simulink model "schema4"  (R2020b)
settings: Solver=VariableStepAuto  StartTime=0.0  StopTime=10.0  RelTol=1e-3
values from neighbouring files (symbols this model uses):
  DenC = [1]    [TP2.m]    (also in ptschema2.m; ptschema3.m)
  DenG = [1/(16.89*50) 1/16.89 0]    [TP2.m]    (also in ptschema2.m = [1/(16.89*50)  1/16.89 0]; ptschema3.m)
  NumC = [1]    [TP2.m]    (also in ptschema2.m; ptschema3.m)
  NumG = [1]    [TP2.m]    (also in ptschema2.m; ptschema3.m)
settings Model: Creator=Antoine  LastModifiedBy=Antoine

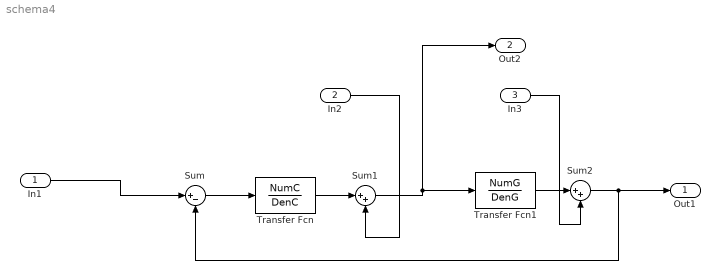
== system schema4 ==
  In1 : Inport
  In2 : Inport  Port=2
  In3 : Inport  Port=3
  Sum : Sum  Inputs=|+-
  Sum1 : Sum  Inputs=|++
  Sum2 : Sum  Inputs=|++
  Transfer Fcn : TransferFcn  Numerator=NumC  Denominator=DenC
  Transfer Fcn1 : TransferFcn  Numerator=NumG  Denominator=DenG
  Out1 : Outport
  Out2 : Outport  Port=2
  wires:
  Sum/1 -> Transfer Fcn/1
  Transfer Fcn/1 -> Sum1/1
  In2/1 -> Sum1/2
  Sum1/1 -> Out2/1, Transfer Fcn1/1
  Transfer Fcn1/1 -> Sum2/1
  Sum2/1 -> Out1/1, Sum/2
  In3/1 -> Sum2/2
  In1/1 -> Sum/1
